simulink model "ControlCalculator"  (R2019b)
settings: Solver=VariableStepAuto  StartTime=0.0  StopTime=5  MaxStep=.01  RelTol=1e-3
libraries: simulink x1, cstblocks x1
settings Model: Creator=mrrya  LastModifiedBy=mrrya
settings SolverCC: ShapePreserveControl=EnableAll

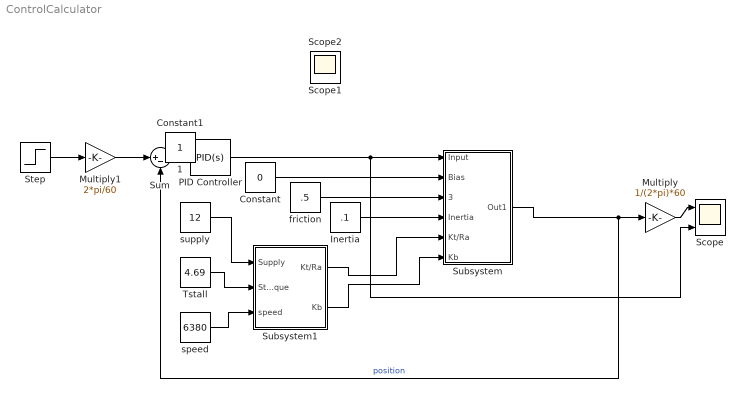
== system ControlCalculator ==
  Constant : Constant  Value=0
  Inertia : Constant  Value=.1
  Multiply : Gain  Gain=1/(2*pi)*60
  Multiply1 : Gain  Gain=2*pi/60
  PID Controller : simulink/Continuous/PID Controller  Controller=PID  Form=Parallel  TimeDomain=Continuous-time  SampleTime=-1  IntegratorMethod=Forward Euler  FilterMethod=Forward Euler  ControllerParametersSource=internal  P=1  I=0  D=.4  UseFilter=on  N=1  TunerSelectOption=Transfer Function Based (PID Tuner App)  InitialConditionSource=internal  InitialConditionForIntegrator=0  InitialConditionForFilter=0  DifferentiatorICPrevScaledInput=0  ExternalReset=none  TrackingMode=off  Kt=1  LimitOutput=off  UpperSaturationLimit=257  LowerSaturationLimit=-257  LinearizeAsGain=on  AntiWindupMode=none  Kb=1  POutMin=[]  POutMax=[]  IOutMin=[]  IOutMax=[]  DOutMin=[]  DOutMax=[]  NOutMin=[]  NOutMax=[]  SumOutMin=[]  SumOutMax=[]  SaturationOutMin=[]  SaturationOutMax=[]  PParamMin=[]  PParamMax=[]  IParamMin=[]  IParamMax=[]  DParamMin=[]  DParamMax=[]  NParamMin=[]  NParamMax=[]  KbParamMin=[]  KbParamMax=[]  KtParamMin=[]  KtParamMax=[]  KbOutMin=[]  KbOutMax=[]  KtOutMin=[]  KtOutMax=[]  IntegratorOutMin=[]  IntegratorOutMax=[]  FilterOutMin=[]  FilterOutMax=[]  SumI1OutMin=[]  SumI1OutMax=[]  SumI2OutMin=[]  SumI2OutMax=[]  SumI3OutMin=[]  SumI3OutMax=[]  SumI4OutMin=[]  SumI4OutMax=[]  SumDOutMin=[]  SumDOutMax=[]  DifferentiatorOutMin=[]  DifferentiatorOutMax=[]  FilterDiffOutCoefMin=[]  FilterDiffOutCoefMax=[]  ReciprocalOutMin=[]  ReciprocalOutMax=[]  SumDenOutMin=[]  SumDenOutMax=[]  SumNumOutMin=[]  SumNumOutMax=[]  DivideOutMin=[]  DivideOutMax=[]  IntegratorContinuousStateAttributes=''  IntegratorStateMustResolveToSignalObject=off  IntegratorRTWStateStorageClass=Auto  FilterContinuousStateAttributes=''  FilterStateMustResolveToSignalObject=off  FilterRTWStateStorageClass=Auto  ParallelPVariant=InternalParameters  IdealPVariant=Disabled  IVariant=InternalParameters  DVariant=InternalParameters  IntegratorVariant=Continuous  SatVariant=Disabled  AWVariant=Passthrough  PCopyVariant=Disabled  TRVariant=Disabled  FdbkBlocksVariant=Forward  IdealPFdbkVariant=Disabled  SatFdbkVariant=Disabled  DerivativeFilterVariant=ContFilter  NVariant=InternalParameters  NCopyVariant=Disabled  FilterICVariant=InternalICsFilter  IntegratorICVariant=InternalICs  ExternalResetVariant=Disabled  TRSumVariant=Passthrough  SumFdbkVariant=Disabled  SumVariant=Sum_PID
  Scope : Scope  NumInputPorts=2
  Step : Step  Time=0  After=5000  SampleTime=0
  Subsystem : Subsystem
  Subsystem1 : Subsystem
  Sum : Sum  Inputs=|+-
  Tstall : Constant  Value=4.69
  friction : Constant  Value=.5
  speed : Constant  Value=6380
  supply : Constant  Value=12
  1 : Constant  IOType=siggen
  Constant1 : Constant  IOType=siggen
  Scope1 : Scope
  Scope2 : Scope
  wires:
  Inertia/1 -> Subsystem/4(Inertia)
  friction/1 -> Subsystem/3(Friction)
  Constant/1 -> Subsystem/2(Bias)
  Subsystem/1(Out1) -> Sum/2, Multiply/1  "position"
  Step/1 -> Multiply1/1
  Sum/1 -> PID Controller/1
  PID Controller/1 -> Scope/2, Subsystem/1(Input)
  Subsystem1/1(Kt/Ra) -> Subsystem/5(Kt/Ra)
  Subsystem1/2(Kb) -> Subsystem/6(Kb)
  supply/1 -> Subsystem1/1(Supply)
  Tstall/1 -> Subsystem1/2(Stall torque)
  speed/1 -> Subsystem1/3(speed)
  Multiply/1 -> Scope/1
  Multiply1/1 -> Sum/1

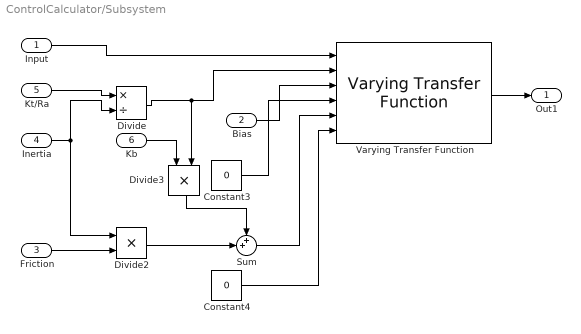
== system ControlCalculator/Subsystem ==
  Input : Inport
  Bias : Inport  Port=2
  Friction : Inport  Port=3
  Inertia : Inport  Port=4
  Kt/Ra : Inport  Port=5
  Kb : Inport  Port=6
  Constant3 : Constant  Value=0
  Constant4 : Constant  Value=0
  Divide : Product  Inputs=*/
  Divide2 : Product  Inputs=**
  Divide3 : Product  Inputs=**
  Sum : Sum  Inputs=++|
  Varying Transfer Function : cstblocks/Linear Parameter Varying/Varying Transfer Function  N=2
      settings: SourceProductName=Control System Toolbox
  Out1 : Outport
  wires:
  Divide3/1 -> Sum/1
  Input/1 -> Varying Transfer Function/1
  Constant3/1 -> Varying Transfer Function/4
  Varying Transfer Function/1 -> Out1/1
  Inertia/1 -> Divide/2, Divide2/1
  Bias/1 -> Varying Transfer Function/3
  Kb/1 -> Divide3/1
  Constant4/1 -> Varying Transfer Function/6
  Sum/1 -> Varying Transfer Function/5
  Divide2/1 -> Sum/2
  Friction/1 -> Divide2/2
  Kt/Ra/1 -> Divide/1
  Divide/1 -> Varying Transfer Function/2, Divide3/2

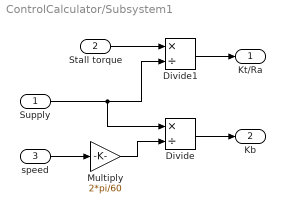
== system ControlCalculator/Subsystem1 ==
  Supply : Inport
  Stall torque : Inport  Port=2
  speed : Inport  Port=3
  Divide : Product  Inputs=*/
  Divide1 : Product  Inputs=*/
  Multiply : Gain  Gain=2*pi/60
  Kt/Ra : Outport
  Kb : Outport  Port=2
  wires:
  Supply/1 -> Divide1/2, Divide/1
  speed/1 -> Multiply/1
  Divide/1 -> Kb/1
  Stall torque/1 -> Divide1/1
  Divide1/1 -> Kt/Ra/1
  Multiply/1 -> Divide/2
